simulink model "mpc_misonoise"  (R2023a)
settings: Solver=ode45  StartTime=0.0  StopTime=145  RelTol=1e-3
values from neighbouring files (symbols this model uses):
  omega = 2*pi/10    (= 0.628318530718)    [mpcmiso1.m]
undefined symbols (not defined in the file or in its folder): A, B, C, D
libraries: mpclib x1
settings Model: ExtModeTrigMode=oneshot  Creator=The MathWorks, Inc.  LastModifiedBy=The MathWorks, Inc.
settings SolverCC: AlgebraicLoopSolver=TrustRegion  MaxZcPerStep=1
settings DataIOCC: SaveFormat=Array  ReturnWorkspaceOutputs=off  SignalLoggingName=sigsOut
settings OptimizationCC: BooleanDataType=off  ExpressionDepthLimit=2147483647  InitFltsAndDblsToZero=on  LifeSpan=inf
settings DebuggingCC: SaveWithParameterizedLinksMsg=none  UnderspecifiedInitializationDetection=Classic  MergeDetectMultiDrivingBlocksExec=none  CheckExecutionContextPreStartOutputMsg=on  SignalResolutionControl=TryResolveAllWithWarning  MultiTaskDSMMsg=warning  MultiTaskCondExecSysMsg=none  IntegerOverflowMsg=none  FcnCallInpInsideContextMsg=warning  UnconnectedInputMsg=warning  UnconnectedOutputMsg=warning  UnconnectedLineMsg=warning  StateNameClashWarn=warning  SFUnexpectedBacktrackingDiag=warning  SFNoUnconditionalDefaultTransitionDiag=warning  SFExecutionAtInitializationDiag=none  IntegerSaturationMsg=none  ArithmeticOperatorsInVariantConditions=warning
settings HardwareCC: ProdBitPerPointer=32  ProdBitPerSizeT=32  ProdBitPerPtrDiffT=32  ProdLargestAtomicFloat=None  ProdIntDivRoundTo=Undefined  ProdEndianess=Unspecified  ProdWordSize=32  ProdHWDeviceType=32-bit Generic  TargetUnknown=on
settings ModelReferenceCC: EnableRefExpFcnMdlSchedulingChecks=on  PropagateSignalLabelsOutOfModel=off
settings SFSimCC: SimUseLocalCustomCode=off  CustomCodeUndefinedFunction=UseInterfaceOnly
settings RTWCC: RTWUseLocalCustomCode=off  DLArmComputeVersion=19.05
settings CodeAppCC: StateflowObjectComments=on
settings GRTTargetCC: TargetFcnLib=ansi_tfl_tmw.mat  TargetLangStandard=C89/C90 (ANSI)  CombineOutputUpdateFcns=off  GRTInterface=on
settings ConfigComp: CovMetricSettings=dw  CovSaveCumulativeToWorkspaceVar=on  CovSaveSingleToWorkspaceVar=on  CovExternalEMLEnable=off  CovSFcnEnable=off

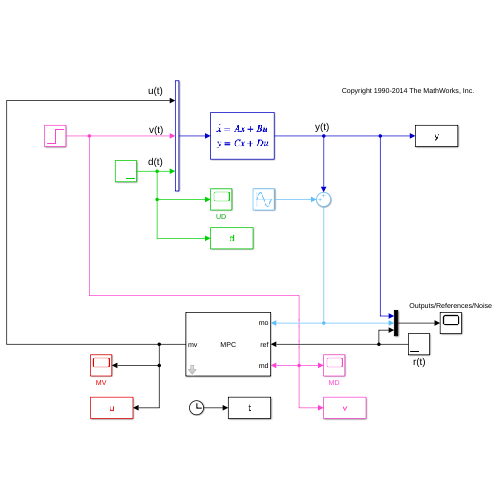
[thumbnail: Simulink's stored preview of the top-level diagram]
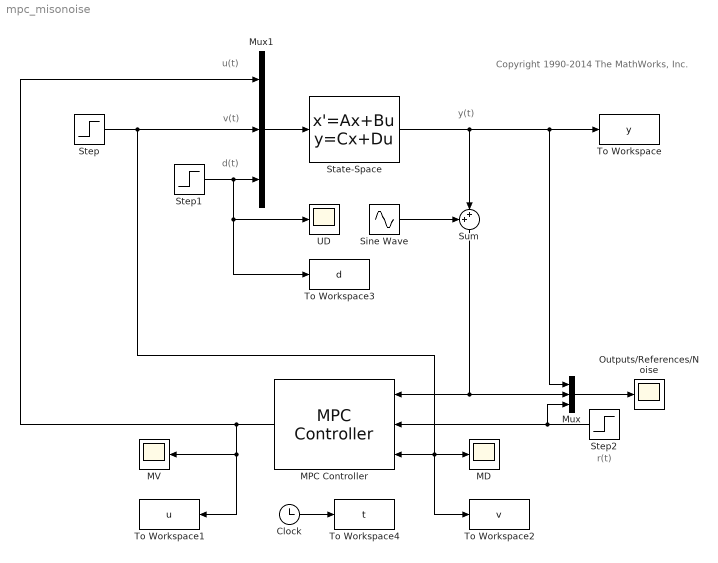
== system mpc_misonoise ==
  note: u(t)
  note: y(t)
  note: r(t)
  note: v(t)
  note: d(t)
  note: Copyright 1990-2014 The MathWorks, Inc.
  Clock : Clock
  MD : Scope
  MPC Controller : mpclib/MPC Controller  mpcobj=mpcobj  x0=[]  is_multiple=0  enable_value=0  return_u0=off  updateMPCinCallerWorkspace=on  md_inport=on  mv_inport=off  uref_inport=off  return_cost=off  return_mvseq=off  return_qpstatus=off  return_xseq=off  return_state=off  return_ovseq=off  state_inport=off  umin_inport=off  umax_inport=off  ymin_inport=off  ymax_inport=off  cc_inport=off  ywt_inport=off  uwt_inport=off  duwt_inport=off  rhoeps_inport=off  pm_inport=off  MaximumP=10  HorizonChoice=FixedHorizon  n_ts=0.2  n_p=40  n_mv=1  n_md=1  n_ud=1  n_mo=1  n_uo=0  BlockDataType=double  SampleTimeInherited=off  switch_inport=off
  MV : Scope
  Mux : Mux  Inputs=3
  Mux1 : Mux  Inputs=3
  Outputs/References/Noise : Scope
  Sine Wave : Sin  Amplitude=.5  Frequency=omega  SampleTime=0
  State-Space : StateSpace  A=A  B=B  C=C  D=D  InitialCondition=[0 0 0 0 0]'
  Step : Step  Time=120  SampleTime=0
  Step1 : Step  Time=60  After=-.5  SampleTime=0
  Step2 : Step  Time=0  SampleTime=0
  Sum : Sum  Inputs=++|  InputSameDT=on  SaturateOnIntegerOverflow=on  OutDataTypeStr=Inherit: Same as first input
  To Workspace : ToWorkspace  VariableName=y  SampleTime=-1
      settings: MaxDataPoints=Inf
  To Workspace1 : ToWorkspace  VariableName=u  SampleTime=-1
      settings: MaxDataPoints=Inf
  To Workspace2 : ToWorkspace  VariableName=v  SampleTime=-1
      settings: MaxDataPoints=Inf
  To Workspace3 : ToWorkspace  VariableName=d  SampleTime=-1
      settings: MaxDataPoints=Inf
  To Workspace4 : ToWorkspace  VariableName=t  SampleTime=-1
      settings: MaxDataPoints=Inf
  UD : Scope
  wires:
  Mux1/1 -> State-Space/1
  Mux/1 -> Outputs/References/Noise/1
  Step1/1 -> Mux1/3, UD/1, To Workspace3/1
  Step/1 -> MD/1, To Workspace2/1, MPC Controller/3, Mux1/2
  MPC Controller/1 -> Mux1/1, MV/1, To Workspace1/1
  State-Space/1 -> Sum/2, To Workspace/1, Mux/1
  Step2/1 -> Mux/3, MPC Controller/2
  Clock/1 -> To Workspace4/1
  Sine Wave/1 -> Sum/1
  Sum/1 -> MPC Controller/1, Mux/2
